simulink model "momentumBasedFlight"  (R2021b)
settings: Solver=VariableStepAuto  StartTime=0.0  StopTime=Config.simulationTime  RelTol=1e-3
InitFcn:
  | cd(fileparts(which(bdroot)));
  | initMomentumBasedFlight;
StopFcn:
  | cd(fileparts(which(bdroot)));
  | stopMomentumBasedFlight;
undefined symbols (not defined in the file or in its folder): aero_config, biasVectorConstraint_feet, Config, ConstraintMatrix_feet, DiscIntNeverNeededParam, frameNames, Frames
libraries: WBToolboxLibrary x104, momentum_flight_control_sublib x4, thrust_estimation_sublib x1, jets_control x1
(part 2 of 3)

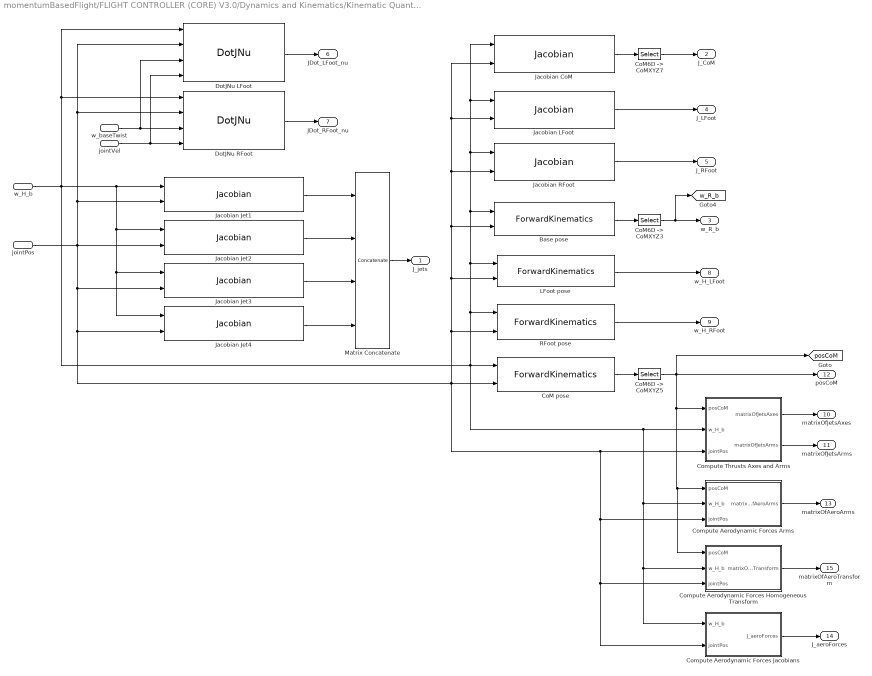
== system momentumBasedFlight/FLIGHT CONTROLLER (CORE) V3.0/Dynamics and Kinematics/Kinematic Quantities ==
  w_H_b : Inport
  jointPos : Inport  Port=2
  w_baseTwist : Inport  Port=3
  jointVel : Inport  Port=4
  Base pose : WBToolboxLibrary/Model/Kinematics/ForwardKinematics  frameName=Frames.BASE_LINK
      settings: SourceProductName=WholeBodyToolbox
  CoM pose : WBToolboxLibrary/Model/Kinematics/ForwardKinematics  frameName=Frames.COM_FRAME
      settings: SourceProductName=WholeBodyToolbox
  "CoM6D -> CoMXYZ3" : Selector  NumberOfDimensions=2  InputPortWidth=7  IndexOptions=Index vector (dialog),Index vector (dialog)  Indices=[1 2 3],[1 2 3]  OutputSizes=1,1
  "CoM6D -> CoMXYZ5" : Selector  NumberOfDimensions=2  InputPortWidth=7  IndexOptions=Index vector (dialog),Index vector (dialog)  Indices=[1 2 3],[4]  OutputSizes=1,1
  "CoM6D -> CoMXYZ7" : Selector  NumberOfDimensions=2  InputPortWidth=7  IndexOptions=Index vector (dialog),Index vector (dialog)  Indices=[1 2 3],[1:6+Config.N_DOF]  OutputSizes=1,1
  Compute Aerodynamic Forces Arms : Subsystem
  Compute Aerodynamic Forces Homogeneous Transform : Subsystem
  Compute Aerodynamic Forces Jacobians : Subsystem
  Compute Thrusts Axes and Arms : Subsystem
  DotJNu LFoot : WBToolboxLibrary/Model/Jacobians/DotJNu  frameName=Frames.LFOOT_FRAME
      settings: SourceProductName=WholeBodyToolbox
  DotJNu RFoot : WBToolboxLibrary/Model/Jacobians/DotJNu  frameName=Frames.RFOOT_FRAME
      settings: SourceProductName=WholeBodyToolbox
  Jacobian CoM : WBToolboxLibrary/Model/Jacobians/Jacobian  frameName=Frames.COM_FRAME
      settings: SourceProductName=WholeBodyToolbox
  Jacobian Jet1 : WBToolboxLibrary/Model/Jacobians/Jacobian  frameName=Frames.JET1_FRAME
      settings: SourceProductName=WholeBodyToolbox
  Jacobian Jet2 : WBToolboxLibrary/Model/Jacobians/Jacobian  frameName=Frames.JET2_FRAME
      settings: SourceProductName=WholeBodyToolbox
  Jacobian Jet3 : WBToolboxLibrary/Model/Jacobians/Jacobian  frameName=Frames.JET3_FRAME
      settings: SourceProductName=WholeBodyToolbox
  Jacobian Jet4 : WBToolboxLibrary/Model/Jacobians/Jacobian  frameName=Frames.JET4_FRAME
      settings: SourceProductName=WholeBodyToolbox
  Jacobian LFoot : WBToolboxLibrary/Model/Jacobians/Jacobian  frameName=Frames.LFOOT_FRAME
      settings: SourceProductName=WholeBodyToolbox
  Jacobian RFoot : WBToolboxLibrary/Model/Jacobians/Jacobian  frameName=Frames.RFOOT_FRAME
      settings: SourceProductName=WholeBodyToolbox
  LFoot pose : WBToolboxLibrary/Model/Kinematics/ForwardKinematics  frameName=Frames.LFOOT_FRAME
      settings: SourceProductName=WholeBodyToolbox
  Matrix Concatenate : Concatenate  NumInputs=4  Mode=Multidimensional array
  RFoot pose : WBToolboxLibrary/Model/Kinematics/ForwardKinematics  frameName=Frames.RFOOT_FRAME
      settings: SourceProductName=WholeBodyToolbox
  J_jets : Outport  VectorParamsAs1DForOutWhenUnconnected=off
  J_CoM : Outport  Port=2  VectorParamsAs1DForOutWhenUnconnected=off
  w_R_b : Outport  Port=3  VectorParamsAs1DForOutWhenUnconnected=off
  J_LFoot : Outport  Port=4  VectorParamsAs1DForOutWhenUnconnected=off
  J_RFoot : Outport  Port=5  VectorParamsAs1DForOutWhenUnconnected=off
  JDot_LFoot_nu : Outport  Port=6  VectorParamsAs1DForOutWhenUnconnected=off
  JDot_RFoot_nu : Outport  Port=7  VectorParamsAs1DForOutWhenUnconnected=off
  w_H_LFoot : Outport  Port=8  VectorParamsAs1DForOutWhenUnconnected=off
  w_H_RFoot : Outport  Port=9  VectorParamsAs1DForOutWhenUnconnected=off
  matrixOfJetsAxes : Outport  Port=10  VectorParamsAs1DForOutWhenUnconnected=off
  matrixOfJetsArms : Outport  Port=11  VectorParamsAs1DForOutWhenUnconnected=off
  posCoM : Outport  Port=12  VectorParamsAs1DForOutWhenUnconnected=off
  matrixOfAeroArms : Outport  Port=13
  J_aeroForces : Outport  Port=14
  matrixOfAeroTransform : Outport  Port=15
  tag scope: posCoM=global, w_R_b=global
  wires:
  "CoM6D -> CoMXYZ7"/1 -> J_CoM/1
  Jacobian Jet4/1 -> Matrix Concatenate/4
  Jacobian Jet3/1 -> Matrix Concatenate/3
  Jacobian Jet2/1 -> Matrix Concatenate/2
  Jacobian Jet1/1 -> Matrix Concatenate/1
  Compute Thrusts Axes and Arms/1(matrixOfJetsAxes) -> matrixOfJetsAxes/1
  Compute Thrusts Axes and Arms/2(matrixOfJetsArms) -> matrixOfJetsArms/1
  Base pose/1 -> "CoM6D -> CoMXYZ3"/1
  LFoot pose/1 -> w_H_LFoot/1
  RFoot pose/1 -> w_H_RFoot/1
  w_baseTwist/1 -> DotJNu RFoot/3, DotJNu LFoot/3
  jointVel/1 -> DotJNu LFoot/4, DotJNu RFoot/4
  DotJNu LFoot/1 -> JDot_LFoot_nu/1
  DotJNu RFoot/1 -> JDot_RFoot_nu/1
  Jacobian LFoot/1 -> J_LFoot/1
  Jacobian RFoot/1 -> J_RFoot/1
  Jacobian CoM/1 -> "CoM6D -> CoMXYZ7"/1
  jointPos/1 -> Jacobian Jet1/2, DotJNu RFoot/2, DotJNu LFoot/2, Jacobian Jet2/2, Base pose/2, Jacobian CoM/2, Jacobian LFoot/2, Jacobian RFoot/2, LFoot pose/2, RFoot pose/2, CoM pose/2, Compute Aerodynamic Forces Homogeneous Transform/3(jointPos), Compute Aerodynamic Forces Jacobians/2(jointPos), Compute Aerodynamic Forces Arms/3(jointPos), Compute Thrusts Axes and Arms/3(jointPos), Jacobian Jet4/2, Jacobian Jet3/2
  "CoM6D -> CoMXYZ3"/1 -> [w_R_b], w_R_b/1
  w_H_b/1 -> Jacobian Jet1/1, Jacobian Jet2/1, Jacobian Jet3/1, Jacobian Jet4/1, DotJNu RFoot/1, DotJNu LFoot/1, Compute Aerodynamic Forces Homogeneous Transform/2(w_H_b), Compute Aerodynamic Forces Jacobians/1(w_H_b), Compute Aerodynamic Forces Arms/2(w_H_b), Compute Thrusts Axes and Arms/2(w_H_b), CoM pose/1, RFoot pose/1, Jacobian RFoot/1, Jacobian CoM/1, Jacobian LFoot/1, Base pose/1, LFoot pose/1
  CoM pose/1 -> "CoM6D -> CoMXYZ5"/1
  Matrix Concatenate/1 -> J_jets/1
  "CoM6D -> CoMXYZ5"/1 -> Compute Aerodynamic Forces Homogeneous Transform/1(posCoM), Compute Aerodynamic Forces Arms/1(posCoM), Compute Thrusts Axes and Arms/1(posCoM), [posCoM], posCoM/1
  Compute Aerodynamic Forces Arms/1(matrixOfAeroArms) -> matrixOfAeroArms/1
  Compute Aerodynamic Forces Jacobians/1(J_aeroForces) -> J_aeroForces/1
  Compute Aerodynamic Forces Homogeneous Transform/1(matrixOfCoMTransform) -> matrixOfAeroTransform/1

== system momentumBasedFlight/FLIGHT CONTROLLER (CORE) V3.0/Estimated or Measured Thrusts/ Thrust Estimator ==
  w_H_b : Inport
  jointPos : Inport  Port=2
  dynamics : Inport  Port=3
  wrench_LFoot : Inport  Port=4
  wrench_RFoot : Inport  Port=5
  throttle : Inport  Port=6
  Enable : EnablePort
  Bus Selector : BusSelector  OutputSignals=L
  Constant : Constant  Value=0
  Constant1 : Constant
  EKF-MOMENTUM_JET_FEET-CMM_FEET : thrust_estimation_sublib/For Simulation/EKF-MOMENTUM_JET_FEET-CMM_FEET  Ts=Config.tStep  Frames=Frames  T0=[0.0; 0.0; 0.0; 0.0]  dot_T0=[0.0; 0.0; 0.0; 0.0]  h0=[0.0; 0.0; 0.0; 0.0; 0.0; 0.0]  fLF0=[0.0; 0.0; 200.0; 0.0; 0.0; 0.0]  fRF0=[0.0; 0.0; 200.0; 0.0; 0.0; 0.0]  P0=blkdiag(eye(4)*1e1, eye(4)*1e1, eye(6)*1e1, eye(6)*1e1, eye(6)*1e1)  Q=blkdiag(eye(4)*1e1, eye(4)*1e1, eye(6)*1e1, eye(6)*1e1, eye(6)*1e1)  R=blkdiag(eye(6)*1e1, eye(6)*1e1, eye(6)*1e1)  jetC_P100=Config.jetC_P100  jetC_P220=Config.jetC_P220
      settings: SourceProductName=iRonCub Library
  Manual Switch : ManualSwitch
  Terminator : Terminator
  Terminator1 : Terminator
  Terminator2 : Terminator
  Unit Delay : UnitDelay  SampleTime=-1  HasFrameUpgradeWarning=on
  jetIntensities_Estimated : Outport
  jetIntensitiesDot_Estimated : Outport  Port=2
  wires:
  Unit Delay/1 -> EKF-MOMENTUM_JET_FEET-CMM_FEET/1
  wrench_RFoot/1 -> EKF-MOMENTUM_JET_FEET-CMM_FEET/6
  wrench_LFoot/1 -> EKF-MOMENTUM_JET_FEET-CMM_FEET/5
  EKF-MOMENTUM_JET_FEET-CMM_FEET/5 -> Terminator2/1
  EKF-MOMENTUM_JET_FEET-CMM_FEET/4 -> Terminator1/1
  EKF-MOMENTUM_JET_FEET-CMM_FEET/3 -> Terminator/1
  jointPos/1 -> EKF-MOMENTUM_JET_FEET-CMM_FEET/2
  w_H_b/1 -> EKF-MOMENTUM_JET_FEET-CMM_FEET/3
  throttle/1 -> Unit Delay/1
  EKF-MOMENTUM_JET_FEET-CMM_FEET/2 -> jetIntensitiesDot_Estimated/1
  EKF-MOMENTUM_JET_FEET-CMM_FEET/1 -> jetIntensities_Estimated/1
  Bus Selector/1 -> EKF-MOMENTUM_JET_FEET-CMM_FEET/4  "<L>"
  dynamics/1 -> Bus Selector/1
  Manual Switch/1 -> EKF-MOMENTUM_JET_FEET-CMM_FEET/7
  Constant/1 -> Manual Switch/2
  Constant1/1 -> Manual Switch/1

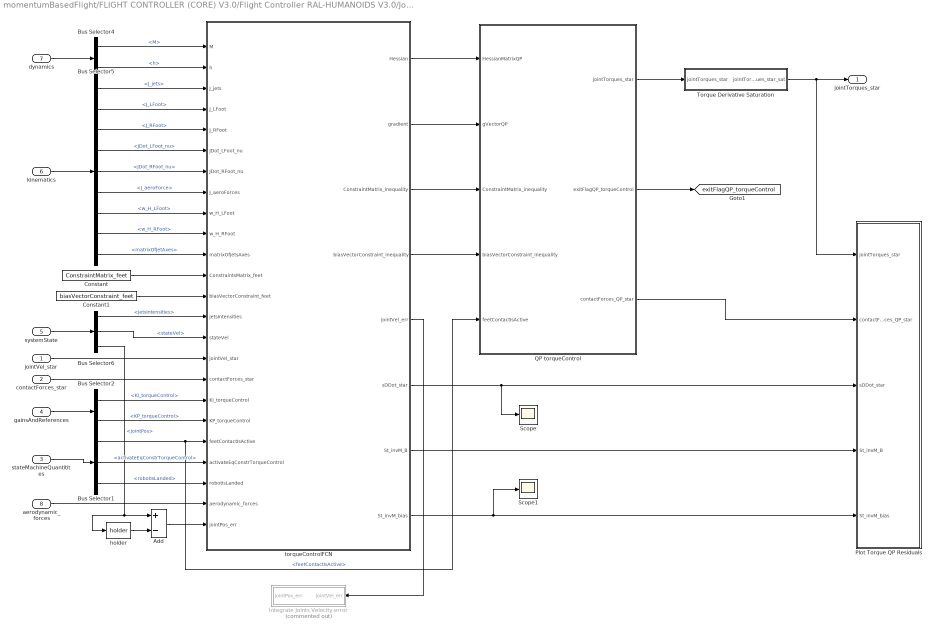
== system momentumBasedFlight/FLIGHT CONTROLLER (CORE) V3.0/Flight Controller RAL-HUMANOIDS V3.0/Joint Torque Control for Flying ==
  jointVel_star : Inport
  contactForces_star : Inport  Port=2
  stateMachineQuantitites : Inport  Port=3
  gainsAndReferences : Inport  Port=4
  systemState : Inport  Port=5
  kinematics : Inport  Port=6
  dynamics : Inport  Port=7
  aerodynamic_forces : Inport  Port=8
  Add : Sum  Inputs=+-
  Bus Selector1 : BusSelector  OutputSignals=feetContactIsActive,activateEqConstrTorqueControl,robotIsLanded
  Bus Selector2 : BusSelector  OutputSignals=KI_torqueControl,KP_torqueControl
  Bus Selector4 : BusSelector  OutputSignals=M,h
  Bus Selector5 : BusSelector  OutputSignals=J_jets,J_LFoot,J_RFoot,JDot_LFoot_nu,JDot_RFoot_nu,J_aeroForce,w_H_LFoot,w_H_RFoot,matrixOfJetAxes
  Bus Selector6 : BusSelector  OutputSignals=jetsIntensities,stateVel,jointPos
  Constant : Constant  Value=ConstraintMatrix_feet
  Constant1 : Constant  Value=biasVectorConstraint_feet
  Integrate Joints Velocity error : Subsystem  Commented=on
  Plot Torque QP Residuals : Subsystem
  QP torqueControl : Subsystem
  Scope : Scope
  Scope1 : Scope
  Torque Derivative Saturation : Subsystem
  "holder " : WBToolboxLibrary/Utilities/holder 
      settings: SourceProductName=WholeBodyToolbox
  torqueControlFCN : MATLAB Function  TreatAsAtomicUnit=on
  jointTorques_star : Outport  VectorParamsAs1DForOutWhenUnconnected=off
  tag scope: exitFlagQP_torqueControl=global
  wires:
  Torque Derivative Saturation/1(jointTorques_star_sat) -> Plot Torque QP Residuals/1(jointTorques_star), jointTorques_star/1
  Bus Selector1/2 -> torqueControlFCN/21(activateEqConstrTorqueControl)  "<activateEqConstrTorqueControl>"
  Bus Selector1/3 -> torqueControlFCN/22(robotIsLanded)  "<robotIsLanded>"
  torqueControlFCN/5(jointVel_err) -> Integrate Joints Velocity error/1(jointVel_err)
  Bus Selector5/9 -> torqueControlFCN/11(matrixOfJetsAxes)  "<matrixOfJetAxes>"
  jointVel_star/1 -> torqueControlFCN/16(jointVel_star)
  torqueControlFCN/4(biasVectorConstraint_inequality) -> QP torqueControl/4(biasVectorConstraint_inequality)
  torqueControlFCN/3(ConstraintMatrix_inequality) -> QP torqueControl/3(ConstraintMatrix_inequality)
  torqueControlFCN/2(gradient) -> QP torqueControl/2(gVectorQP)
  torqueControlFCN/1(Hessian) -> QP torqueControl/1(HessianMatrixQP)
  Bus Selector2/2 -> torqueControlFCN/19(KP_torqueControl)  "<KP_torqueControl>"
  Bus Selector2/1 -> torqueControlFCN/18(KI_torqueControl)  "<KI_torqueControl>"
  gainsAndReferences/1 -> Bus Selector2/1
  Bus Selector1/1 -> QP torqueControl/5(feetContactIsActive), torqueControlFCN/20(feetContactIsActive)  "<feetContactIsActive>"
  stateMachineQuantitites/1 -> Bus Selector1/1
  Bus Selector6/1 -> torqueControlFCN/14(jetsIntensities)  "<jetsIntensities>"
  QP torqueControl/2(exitFlagQP_torqueControl) -> [exitFlagQP_torqueControl]
  QP torqueControl/1(jointTorques_star) -> Torque Derivative Saturation/1(jointTorques_star)
  contactForces_star/1 -> torqueControlFCN/17(contactForces_star)
  Constant/1 -> torqueControlFCN/12(ConstraintsMatrix_feet)
  Constant1/1 -> torqueControlFCN/13(biasVectorConstraint_feet)
  Bus Selector5/8 -> torqueControlFCN/10(w_H_RFoot)  "<w_H_RFoot>"
  Bus Selector5/7 -> torqueControlFCN/9(w_H_LFoot)  "<w_H_LFoot>"
  Bus Selector5/5 -> torqueControlFCN/7(JDot_RFoot_nu)  "<JDot_RFoot_nu>"
  Bus Selector5/4 -> torqueControlFCN/6(JDot_LFoot_nu)  "<JDot_LFoot_nu>"
  Bus Selector5/3 -> torqueControlFCN/5(J_RFoot)  "<J_RFoot>"
  Bus Selector5/2 -> torqueControlFCN/4(J_LFoot)  "<J_LFoot>"
  Bus Selector5/1 -> torqueControlFCN/3(J_jets)  "<J_jets>"
  Bus Selector4/2 -> torqueControlFCN/2(h)  "<h>"
  Bus Selector4/1 -> torqueControlFCN/1(M)  "<M>"
  kinematics/1 -> Bus Selector5/1
  systemState/1 -> Bus Selector6/1
  dynamics/1 -> Bus Selector4/1
  Bus Selector6/2 -> torqueControlFCN/15(stateVel)  "<stateVel>"
  Bus Selector5/6 -> torqueControlFCN/8(J_aeroForces)  "<J_aeroForce>"
  aerodynamic_forces/1 -> torqueControlFCN/23(aerodynamic_forces)
  Bus Selector6/3 -> "holder "/1, Add/1  "<jointPos>"
  Add/1 -> torqueControlFCN/24(jointPos_err)
  "holder "/1 -> Add/2
  QP torqueControl/3(contactForces_QP_star) -> Plot Torque QP Residuals/2(contactForces_QP_star)
  torqueControlFCN/6(sDDot_star) -> Scope/1, Plot Torque QP Residuals/3(sDDot_star)
  torqueControlFCN/7(St_invM_B) -> Plot Torque QP Residuals/4(St_invM_B)
  torqueControlFCN/8(St_invM_bias) -> Scope1/1, Plot Torque QP Residuals/5(St_invM_bias)

== system momentumBasedFlight/FLIGHT CONTROLLER (CORE) V3.0/Flight Controller RAL-HUMANOIDS V3.0/Momentum Control for Flying ==
  stateMachineQuantitites : Inport
  gainsAndReferences : Inport  Port=2
  systemState : Inport  Port=3
  kinematics : Inport  Port=4
  dynamics : Inport  Port=5
  aerodynamic_forces : Inport  Port=6
  Momentum Control : Subsystem
  QP Solver and Integrate Contact Forces Derivative : Subsystem
  jointVel_star : Outport  VectorParamsAs1DForOutWhenUnconnected=off
  contactForces_star : Outport  Port=2  VectorParamsAs1DForOutWhenUnconnected=off
  jetsIntensitiesDot_star : Outport  Port=3  VectorParamsAs1DForOutWhenUnconnected=off
  wires:
  QP Solver and Integrate Contact Forces Derivative/3(jointVel_star) -> jointVel_star/1
  QP Solver and Integrate Contact Forces Derivative/1(contactForces_star) -> Momentum Control/1(contactForces_hat), contactForces_star/1  "WARNING! estimated contact forces are assumed to be coincident with contactForces_star"
  Momentum Control/4(uppeBoundQP) -> QP Solver and Integrate Contact Forces Derivative/4(upperBoundQP)
  Momentum Control/3(lowerBoundQP) -> QP Solver and Integrate Contact Forces Derivative/3(lowerBoundQP)
  Momentum Control/2(gVectorQP) -> QP Solver and Integrate Contact Forces Derivative/2(gVectorQP)
  Momentum Control/1(HessianMatrixQP) -> QP Solver and Integrate Contact Forces Derivative/1(HessianMatrixQP)
  stateMachineQuantitites/1 -> QP Solver and Integrate Contact Forces Derivative/5(stateMachineQuantities), Momentum Control/6(stateMachineQuantitites)
  gainsAndReferences/1 -> Momentum Control/5(gainsAndReferences)
  dynamics/1 -> Momentum Control/4(dynamics), QP Solver and Integrate Contact Forces Derivative/7(dynamics)
  kinematics/1 -> Momentum Control/3(kinematics)
  systemState/1 -> QP Solver and Integrate Contact Forces Derivative/6(systemState), Momentum Control/2(systemState)
  QP Solver and Integrate Contact Forces Derivative/2(jetsIntensitiesDot_star) -> jetsIntensitiesDot_star/1
  aerodynamic_forces/1 -> Momentum Control/7(aerodynamic_forces)

== system momentumBasedFlight/FLIGHT CONTROLLER (CORE) V3.0/Flight Controller RAL-HUMANOIDS V3.0/deadZone ==
  u : Inport
  Constant : Constant  Value=Config.sat.deadZoneThresholdJointVel
  Deadzone Function : MATLAB Function  TreatAsAtomicUnit=on
  u_cut : Outport  VectorParamsAs1DForOutWhenUnconnected=off
  wires:
  Constant/1 -> Deadzone Function/2(thr)
  u/1 -> Deadzone Function/1(u)
  Deadzone Function/1(y) -> u_cut/1

== system momentumBasedFlight/FLOATING BASE ESTIMATOR/Compute State Velocity/Feet Jacobians ==
  jointPos : Inport
  w_H_b : Inport  Port=2
  Jacobian l_sole : WBToolboxLibrary/Model/Jacobians/Jacobian  frameName=Frames.LFOOT_FRAME
      settings: SourceProductName=WholeBodyToolbox
  Jacobian r_sole : WBToolboxLibrary/Model/Jacobians/Jacobian  frameName=Frames.RFOOT_FRAME
      settings: SourceProductName=WholeBodyToolbox
  J_l_sole : Outport  VectorParamsAs1DForOutWhenUnconnected=off
  J_r_sole : Outport  Port=2  VectorParamsAs1DForOutWhenUnconnected=off
  wires:
  Jacobian l_sole/1 -> J_l_sole/1
  Jacobian r_sole/1 -> J_r_sole/1
  w_H_b/1 -> Jacobian r_sole/1, Jacobian l_sole/1
  jointPos/1 -> Jacobian l_sole/2, Jacobian r_sole/2

== system momentumBasedFlight/FLOATING BASE ESTIMATOR/Compute base to fixed link transform/LFoot to base link transform  ==
  jointPos : Inport
  inertial : Inport  Port=2
  w_H_link : Inport  Port=3
  w_H_base_fixed : Inport  Port=4
  Fixed base to imu transform : WBToolboxLibrary/Model/Kinematics/ForwardKinematics  frameName=Frames.IMU
      settings: SourceProductName=WholeBodyToolbox
  Fixed base to root link transform : WBToolboxLibrary/Model/Kinematics/ForwardKinematics  frameName=Frames.BASE_LINK
      settings: SourceProductName=WholeBodyToolbox
  Get Base Rotation From IMU : MATLAB Function  TreatAsAtomicUnit=on
  Inv : Product  Inputs=/*  Multiplication=Matrix(*)
  Inv_2 : Product  Inputs=/*  Multiplication=Matrix(*)
  Neck Position : WBToolboxLibrary/Utilities/YarpRead  portName=Ports.NECK_POS  signalSize=Ports.NECK_POS_PORT_SIZE  timeout=0.5  blocking=off  timestamp=off  autoconnect=on  errorOnConnection=off
      settings: SourceProductName=WholeBodyToolbox
  Selector1 : Selector  InputPortWidth=Ports.IMU_PORT_SIZE  IndexOptions=Index vector (dialog)  Indices=Ports.IMU_PORT_ORIENTATION_INDEX  OutputSizes=1
  Selector2 : Selector  InputPortWidth=Ports.IMU_PORT_SIZE  IndexOptions=Index vector (dialog)  Indices=Ports.IMU_PORT_ORIENTATION_INDEX  OutputSizes=1
  Switch6 : Switch  Criteria=u2 > Threshold
  USE_IMU4EST_BASE : Constant  Value=Config.USE_IMU4EST_BASE
  holder 1 : WBToolboxLibrary/Utilities/holder 
      settings: SourceProductName=WholeBodyToolbox
  holder 2 : WBToolboxLibrary/Utilities/holder 
      settings: SourceProductName=WholeBodyToolbox
  neck transform : Subsystem
  link_H_b : Outport  VectorParamsAs1DForOutWhenUnconnected=off
  wires:
  Switch6/1 -> link_H_b/1
  Inv_2/1 -> Switch6/3, Get Base Rotation From IMU/3(fixedLink_H_base)  "link_H_root"
  USE_IMU4EST_BASE/1 -> Switch6/2
  Inv/1 -> Get Base Rotation From IMU/1(imu_H_fixedLink), holder 1/1  "imu_H_link"
  holder 2/1 -> Selector2/1
  Fixed base to imu transform/1 -> Inv/1
  jointPos/1 -> Fixed base to imu transform/2, Fixed base to root link transform/2
  Get Base Rotation From IMU/1(w_H_b) -> Switch6/1
  Fixed base to root link transform/1 -> Inv_2/2
  inertial/1 -> holder 2/1, Selector1/1
  Neck Position/1 -> neck transform/1(neck port)
  neck transform/1(neck position) -> Get Base Rotation From IMU/6(neck_pos)
  w_H_link/1 -> Inv_2/1, Inv/2
  w_H_base_fixed/1 -> Fixed base to root link transform/1, Fixed base to imu transform/1
  Selector2/1 -> Get Base Rotation From IMU/4(rpyFromIMU_0)
  holder 1/1 -> Get Base Rotation From IMU/2(imu_H_fixedLink_0)
  Selector1/1 -> Get Base Rotation From IMU/5(rpyFromIMU)

== system momentumBasedFlight/FLOATING BASE ESTIMATOR/Compute base to fixed link transform/RFoot to base link transform ==
  jointPos : Inport
  inertial : Inport  Port=2
  w_H_link : Inport  Port=3
  w_H_base_fixed : Inport  Port=4
  Fixed base to imu transform : WBToolboxLibrary/Model/Kinematics/ForwardKinematics  frameName=Frames.IMU
      settings: SourceProductName=WholeBodyToolbox
  Fixed base to root link transform : WBToolboxLibrary/Model/Kinematics/ForwardKinematics  frameName=Frames.BASE_LINK
      settings: SourceProductName=WholeBodyToolbox
  Get Base Rotation From IMU : MATLAB Function  TreatAsAtomicUnit=on
  Inv : Product  Inputs=/*  Multiplication=Matrix(*)
  Inv_2 : Product  Inputs=/*  Multiplication=Matrix(*)
  Neck Position : WBToolboxLibrary/Utilities/YarpRead  portName=Ports.NECK_POS  signalSize=Ports.NECK_POS_PORT_SIZE  timeout=0.5  blocking=off  timestamp=off  autoconnect=on  errorOnConnection=off
      settings: SourceProductName=WholeBodyToolbox
  Selector1 : Selector  InputPortWidth=Ports.IMU_PORT_SIZE  IndexOptions=Index vector (dialog)  Indices=Ports.IMU_PORT_ORIENTATION_INDEX  OutputSizes=1
  Selector2 : Selector  InputPortWidth=Ports.IMU_PORT_SIZE  IndexOptions=Index vector (dialog)  Indices=Ports.IMU_PORT_ORIENTATION_INDEX  OutputSizes=1
  Switch6 : Switch  Criteria=u2 > Threshold
  USE_IMU4EST_BASE : Constant  Value=Config.USE_IMU4EST_BASE
  holder 1 : WBToolboxLibrary/Utilities/holder 
      settings: SourceProductName=WholeBodyToolbox
  holder 2 : WBToolboxLibrary/Utilities/holder 
      settings: SourceProductName=WholeBodyToolbox
  neck transform : Subsystem
  link_H_b : Outport  VectorParamsAs1DForOutWhenUnconnected=off
  wires:
  Switch6/1 -> link_H_b/1
  Inv_2/1 -> Switch6/3, Get Base Rotation From IMU/3(fixedLink_H_base)  "link_H_root"
  USE_IMU4EST_BASE/1 -> Switch6/2
  Inv/1 -> Get Base Rotation From IMU/1(imu_H_fixedLink), holder 1/1  "imu_H_link"
  holder 2/1 -> Selector2/1
  Fixed base to imu transform/1 -> Inv/1
  jointPos/1 -> Fixed base to imu transform/2, Fixed base to root link transform/2
  Get Base Rotation From IMU/1(w_H_b) -> Switch6/1
  Fixed base to root link transform/1 -> Inv_2/2
  inertial/1 -> holder 2/1, Selector1/1
  Neck Position/1 -> neck transform/1(neck port)
  neck transform/1(neck position) -> Get Base Rotation From IMU/6(neck_pos)
  w_H_link/1 -> Inv_2/1, Inv/2
  w_H_base_fixed/1 -> Fixed base to root link transform/1, Fixed base to imu transform/1
  Selector2/1 -> Get Base Rotation From IMU/4(rpyFromIMU_0)
  holder 1/1 -> Get Base Rotation From IMU/2(imu_H_fixedLink_0)
  Selector1/1 -> Get Base Rotation From IMU/5(rpyFromIMU)

== system momentumBasedFlight/Visualizer/Task and Base Frame Kinematics/Combine Rotations ==
  roll : Inport
  pitch : Inport  Port=2
  yaw : Inport  Port=3
  roll_des : Inport  Port=4
  pitch_des : Inport  Port=5
  yaw_des : Inport  Port=6
  Mux : Mux  Inputs=2
  Mux1 : Mux  Inputs=2
  Mux2 : Mux  Inputs=2
  Task rotation combined : Scope  NumInputPorts=3
  wires:
  yaw_des/1 -> Mux2/2
  pitch_des/1 -> Mux1/2
  pitch/1 -> Mux1/1
  roll/1 -> Mux/1
  yaw/1 -> Mux2/1
  roll_des/1 -> Mux/2
  Mux2/1 -> Task rotation combined/3
  Mux1/1 -> Task rotation combined/2
  Mux/1 -> Task rotation combined/1

== system momentumBasedFlight/FLIGHT CONTROLLER (CORE) V3.0/Dynamics and Kinematics/Dynamic Quantities/Compute Centroidal Inertia ==
  M : Inport
  w_H_b : Inport  Port=2
  posCoM : Inport  Port=3
  Compute Centroidal Inertia : MATLAB Function  TreatAsAtomicUnit=on
  Selector : Selector  NumberOfDimensions=2  InputPortWidth=3  IndexOptions=Index vector (dialog),Index vector (dialog)  Indices=[1 2 3],4  OutputSizes=1,1
  w_I_c : Outport  VectorParamsAs1DForOutWhenUnconnected=off
  wires:
  Compute Centroidal Inertia/1(w_I_c) -> w_I_c/1
  posCoM/1 -> Compute Centroidal Inertia/2(posCoM)
  Selector/1 -> Compute Centroidal Inertia/3(posBase)
  w_H_b/1 -> Selector/1
  M/1 -> Compute Centroidal Inertia/1(M)

== system momentumBasedFlight/FLIGHT CONTROLLER (CORE) V3.0/Dynamics and Kinematics/Dynamic Quantities/Momentum and CentroidalMomentum Matrix ==
  w_H_b : Inport
  jointPos : Inport  Port=2
  w_baseTwist : Inport  Port=3
  jointVel : Inport  Port=4
  CentroidalMomentum : WBToolboxLibrary/Model/Dynamics/CentroidalMomentum
      settings: SourceProductName=WholeBodyToolbox
  CentroidalTotalMomentumMatrix : WBToolboxLibrary/Model/Jacobians/CentroidalTotalMomentumMatrix
      settings: SourceProductName=WholeBodyToolbox
  L : Outport  VectorParamsAs1DForOutWhenUnconnected=off
  CMM : Outport  Port=2  VectorParamsAs1DForOutWhenUnconnected=off
  wires:
  CentroidalTotalMomentumMatrix/1 -> CMM/1
  jointVel/1 -> CentroidalMomentum/4
  jointPos/1 -> CentroidalMomentum/2, CentroidalTotalMomentumMatrix/2
  w_H_b/1 -> CentroidalMomentum/1, CentroidalTotalMomentumMatrix/1
  CentroidalMomentum/1 -> L/1
  w_baseTwist/1 -> CentroidalMomentum/3

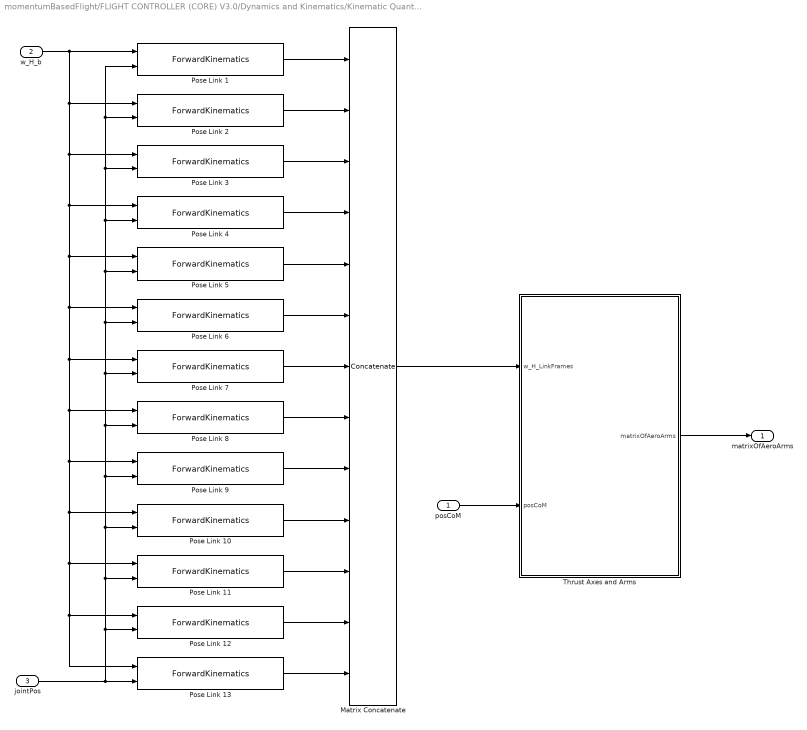
== system momentumBasedFlight/FLIGHT CONTROLLER (CORE) V3.0/Dynamics and Kinematics/Kinematic Quantities/Compute Aerodynamic Forces Arms ==
  posCoM : Inport
  w_H_b : Inport  Port=2
  jointPos : Inport  Port=3
  Matrix Concatenate : Concatenate  NumInputs=13  Mode=Multidimensional array  ConcatenateDimension=2
  Pose Link 1 : WBToolboxLibrary/Model/Kinematics/ForwardKinematics  frameName=frameNames{1}
      settings: SourceProductName=WholeBodyToolbox
  Pose Link 10 : WBToolboxLibrary/Model/Kinematics/ForwardKinematics  frameName=frameNames{10}
      settings: SourceProductName=WholeBodyToolbox
  Pose Link 11 : WBToolboxLibrary/Model/Kinematics/ForwardKinematics  frameName=frameNames{11}
      settings: SourceProductName=WholeBodyToolbox
  Pose Link 12 : WBToolboxLibrary/Model/Kinematics/ForwardKinematics  frameName=frameNames{12}
      settings: SourceProductName=WholeBodyToolbox
  Pose Link 13 : WBToolboxLibrary/Model/Kinematics/ForwardKinematics  frameName=frameNames{13}
      settings: SourceProductName=WholeBodyToolbox
  Pose Link 2 : WBToolboxLibrary/Model/Kinematics/ForwardKinematics  frameName=frameNames{2}
      settings: SourceProductName=WholeBodyToolbox
  Pose Link 3 : WBToolboxLibrary/Model/Kinematics/ForwardKinematics  frameName=frameNames{3}
      settings: SourceProductName=WholeBodyToolbox
  Pose Link 4 : WBToolboxLibrary/Model/Kinematics/ForwardKinematics  frameName=frameNames{4}
      settings: SourceProductName=WholeBodyToolbox
  Pose Link 5 : WBToolboxLibrary/Model/Kinematics/ForwardKinematics  frameName=frameNames{5}
      settings: SourceProductName=WholeBodyToolbox
  Pose Link 6 : WBToolboxLibrary/Model/Kinematics/ForwardKinematics  frameName=frameNames{6}
      settings: SourceProductName=WholeBodyToolbox
  Pose Link 7 : WBToolboxLibrary/Model/Kinematics/ForwardKinematics  frameName=frameNames{7}
      settings: SourceProductName=WholeBodyToolbox
  Pose Link 8 : WBToolboxLibrary/Model/Kinematics/ForwardKinematics  frameName=frameNames{8}
      settings: SourceProductName=WholeBodyToolbox
  Pose Link 9 : WBToolboxLibrary/Model/Kinematics/ForwardKinematics  frameName=frameNames{9}
      settings: SourceProductName=WholeBodyToolbox
  Thrust Axes and Arms : MATLAB Function  TreatAsAtomicUnit=on
  matrixOfAeroArms : Outport  VectorParamsAs1DForOutWhenUnconnected=off
  wires:
  posCoM/1 -> Thrust Axes and Arms/2(posCoM)
  w_H_b/1 -> Pose Link 1/1, Pose Link 4/1, Pose Link 5/1, Pose Link 6/1, Pose Link 7/1, Pose Link 9/1, Pose Link 10/1, Pose Link 11/1, Pose Link 12/1, Pose Link 13/1, Pose Link 8/1, Pose Link 3/1, Pose Link 2/1
  Thrust Axes and Arms/1(matrixOfAeroArms) -> matrixOfAeroArms/1
  jointPos/1 -> Pose Link 13/2, Pose Link 12/2, Pose Link 11/2, Pose Link 10/2, Pose Link 9/2, Pose Link 8/2, Pose Link 7/2, Pose Link 6/2, Pose Link 5/2, Pose Link 4/2, Pose Link 3/2, Pose Link 2/2, Pose Link 1/2
  Matrix Concatenate/1 -> Thrust Axes and Arms/1(w_H_LinkFrames)
  Pose Link 13/1 -> Matrix Concatenate/13
  Pose Link 12/1 -> Matrix Concatenate/12
  Pose Link 11/1 -> Matrix Concatenate/11
  Pose Link 10/1 -> Matrix Concatenate/10
  Pose Link 9/1 -> Matrix Concatenate/9
  Pose Link 8/1 -> Matrix Concatenate/8
  Pose Link 7/1 -> Matrix Concatenate/7
  Pose Link 6/1 -> Matrix Concatenate/6
  Pose Link 5/1 -> Matrix Concatenate/5
  Pose Link 4/1 -> Matrix Concatenate/4
  Pose Link 3/1 -> Matrix Concatenate/3
  Pose Link 2/1 -> Matrix Concatenate/2
  Pose Link 1/1 -> Matrix Concatenate/1

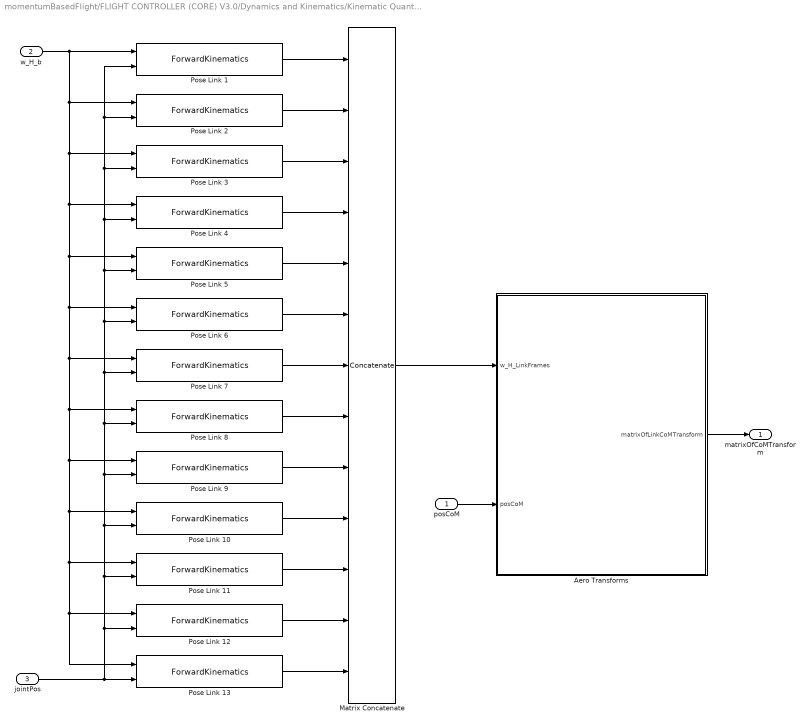
== system momentumBasedFlight/FLIGHT CONTROLLER (CORE) V3.0/Dynamics and Kinematics/Kinematic Quantities/Compute Aerodynamic Forces Homogeneous Transform ==
  posCoM : Inport
  w_H_b : Inport  Port=2
  jointPos : Inport  Port=3
  Aero Transforms : MATLAB Function  TreatAsAtomicUnit=on
  Matrix Concatenate : Concatenate  NumInputs=13  Mode=Multidimensional array  ConcatenateDimension=2
  Pose Link 1 : WBToolboxLibrary/Model/Kinematics/ForwardKinematics  frameName=frameNames{1}
      settings: SourceProductName=WholeBodyToolbox
  Pose Link 10 : WBToolboxLibrary/Model/Kinematics/ForwardKinematics  frameName=frameNames{10}
      settings: SourceProductName=WholeBodyToolbox
  Pose Link 11 : WBToolboxLibrary/Model/Kinematics/ForwardKinematics  frameName=frameNames{11}
      settings: SourceProductName=WholeBodyToolbox
  Pose Link 12 : WBToolboxLibrary/Model/Kinematics/ForwardKinematics  frameName=frameNames{12}
      settings: SourceProductName=WholeBodyToolbox
  Pose Link 13 : WBToolboxLibrary/Model/Kinematics/ForwardKinematics  frameName=frameNames{13}
      settings: SourceProductName=WholeBodyToolbox
  Pose Link 2 : WBToolboxLibrary/Model/Kinematics/ForwardKinematics  frameName=frameNames{2}
      settings: SourceProductName=WholeBodyToolbox
  Pose Link 3 : WBToolboxLibrary/Model/Kinematics/ForwardKinematics  frameName=frameNames{3}
      settings: SourceProductName=WholeBodyToolbox
  Pose Link 4 : WBToolboxLibrary/Model/Kinematics/ForwardKinematics  frameName=frameNames{4}
      settings: SourceProductName=WholeBodyToolbox
  Pose Link 5 : WBToolboxLibrary/Model/Kinematics/ForwardKinematics  frameName=frameNames{5}
      settings: SourceProductName=WholeBodyToolbox
  Pose Link 6 : WBToolboxLibrary/Model/Kinematics/ForwardKinematics  frameName=frameNames{6}
      settings: SourceProductName=WholeBodyToolbox
  Pose Link 7 : WBToolboxLibrary/Model/Kinematics/ForwardKinematics  frameName=frameNames{7}
      settings: SourceProductName=WholeBodyToolbox
  Pose Link 8 : WBToolboxLibrary/Model/Kinematics/ForwardKinematics  frameName=frameNames{8}
      settings: SourceProductName=WholeBodyToolbox
  Pose Link 9 : WBToolboxLibrary/Model/Kinematics/ForwardKinematics  frameName=frameNames{9}
      settings: SourceProductName=WholeBodyToolbox
  matrixOfCoMTransform : Outport  VectorParamsAs1DForOutWhenUnconnected=off
  wires:
  posCoM/1 -> Aero Transforms/2(posCoM)
  w_H_b/1 -> Pose Link 1/1, Pose Link 4/1, Pose Link 5/1, Pose Link 6/1, Pose Link 7/1, Pose Link 9/1, Pose Link 10/1, Pose Link 11/1, Pose Link 12/1, Pose Link 13/1, Pose Link 8/1, Pose Link 3/1, Pose Link 2/1
  Aero Transforms/1(matrixOfLinkCoMTransform) -> matrixOfCoMTransform/1
  jointPos/1 -> Pose Link 13/2, Pose Link 12/2, Pose Link 11/2, Pose Link 10/2, Pose Link 9/2, Pose Link 8/2, Pose Link 7/2, Pose Link 6/2, Pose Link 5/2, Pose Link 4/2, Pose Link 3/2, Pose Link 2/2, Pose Link 1/2
  Matrix Concatenate/1 -> Aero Transforms/1(w_H_LinkFrames)
  Pose Link 13/1 -> Matrix Concatenate/13
  Pose Link 12/1 -> Matrix Concatenate/12
  Pose Link 11/1 -> Matrix Concatenate/11
  Pose Link 10/1 -> Matrix Concatenate/10
  Pose Link 9/1 -> Matrix Concatenate/9
  Pose Link 8/1 -> Matrix Concatenate/8
  Pose Link 7/1 -> Matrix Concatenate/7
  Pose Link 6/1 -> Matrix Concatenate/6
  Pose Link 5/1 -> Matrix Concatenate/5
  Pose Link 4/1 -> Matrix Concatenate/4
  Pose Link 3/1 -> Matrix Concatenate/3
  Pose Link 2/1 -> Matrix Concatenate/2
  Pose Link 1/1 -> Matrix Concatenate/1

== system momentumBasedFlight/FLIGHT CONTROLLER (CORE) V3.0/Dynamics and Kinematics/Kinematic Quantities/Compute Aerodynamic Forces Jacobians ==
  w_H_b : Inport
  jointPos : Inport  Port=2
  Jacobian Link frame 1 : WBToolboxLibrary/Model/Jacobians/Jacobian  frameName=frameNames{1}
      settings: SourceProductName=WholeBodyToolbox
  Jacobian Link frame 10 : WBToolboxLibrary/Model/Jacobians/Jacobian  frameName=frameNames{10}
      settings: SourceProductName=WholeBodyToolbox
  Jacobian Link frame 11 : WBToolboxLibrary/Model/Jacobians/Jacobian  frameName=frameNames{11}
      settings: SourceProductName=WholeBodyToolbox
  Jacobian Link frame 12 : WBToolboxLibrary/Model/Jacobians/Jacobian  frameName=frameNames{12}
      settings: SourceProductName=WholeBodyToolbox
  Jacobian Link frame 13 : WBToolboxLibrary/Model/Jacobians/Jacobian  frameName=frameNames{13}
      settings: SourceProductName=WholeBodyToolbox
  Jacobian Link frame 2 : WBToolboxLibrary/Model/Jacobians/Jacobian  frameName=frameNames{2}
      settings: SourceProductName=WholeBodyToolbox
  Jacobian Link frame 3 : WBToolboxLibrary/Model/Jacobians/Jacobian  frameName=frameNames{3}
      settings: SourceProductName=WholeBodyToolbox
  Jacobian Link frame 4 : WBToolboxLibrary/Model/Jacobians/Jacobian  frameName=frameNames{4}
      settings: SourceProductName=WholeBodyToolbox
  Jacobian Link frame 5 : WBToolboxLibrary/Model/Jacobians/Jacobian  frameName=frameNames{5}
      settings: SourceProductName=WholeBodyToolbox
  Jacobian Link frame 6 : WBToolboxLibrary/Model/Jacobians/Jacobian  frameName=frameNames{6}
      settings: SourceProductName=WholeBodyToolbox
  Jacobian Link frame 7 : WBToolboxLibrary/Model/Jacobians/Jacobian  frameName=frameNames{7}
      settings: SourceProductName=WholeBodyToolbox
  Jacobian Link frame 8 : WBToolboxLibrary/Model/Jacobians/Jacobian  frameName=frameNames{8}
      settings: SourceProductName=WholeBodyToolbox
  Jacobian Link frame 9 : WBToolboxLibrary/Model/Jacobians/Jacobian  frameName=frameNames{9}
      settings: SourceProductName=WholeBodyToolbox
  Matrix Concatenate : Concatenate  NumInputs=13  Mode=Multidimensional array
  compute matrix of link CoM Jacobians : MATLAB Function  TreatAsAtomicUnit=on
  J_aeroForces : Outport  VectorParamsAs1DForOutWhenUnconnected=off
  wires:
  w_H_b/1 -> Jacobian Link frame 1/1, Jacobian Link frame 2/1, Jacobian Link frame 3/1, Jacobian Link frame 4/1, Jacobian Link frame 5/1, Jacobian Link frame 6/1, Jacobian Link frame 7/1, Jacobian Link frame 8/1, Jacobian Link frame 9/1, Jacobian Link frame 10/1, Jacobian Link frame 11/1, Jacobian Link frame 13/1, Jacobian Link frame 12/1, compute matrix of link CoM Jacobians/1(w_H_b)
  jointPos/1 -> Jacobian Link frame 13/2, Jacobian Link frame 12/2, Jacobian Link frame 11/2, Jacobian Link frame 10/2, Jacobian Link frame 9/2, Jacobian Link frame 8/2, Jacobian Link frame 7/2, Jacobian Link frame 6/2, Jacobian Link frame 5/2, Jacobian Link frame 4/2, Jacobian Link frame 3/2, Jacobian Link frame 1/2, Jacobian Link frame 2/2
  Jacobian Link frame 1/1 -> Matrix Concatenate/1
  Jacobian Link frame 2/1 -> Matrix Concatenate/2
  Jacobian Link frame 3/1 -> Matrix Concatenate/3
  Jacobian Link frame 5/1 -> Matrix Concatenate/5
  Jacobian Link frame 4/1 -> Matrix Concatenate/4
  Jacobian Link frame 6/1 -> Matrix Concatenate/6
  Jacobian Link frame 7/1 -> Matrix Concatenate/7
  Jacobian Link frame 8/1 -> Matrix Concatenate/8
  Jacobian Link frame 9/1 -> Matrix Concatenate/9
  Jacobian Link frame 10/1 -> Matrix Concatenate/10
  Jacobian Link frame 11/1 -> Matrix Concatenate/11
  Jacobian Link frame 12/1 -> Matrix Concatenate/12
  Jacobian Link frame 13/1 -> Matrix Concatenate/13
  compute matrix of link CoM Jacobians/1(J_aeroForces) -> J_aeroForces/1
  Matrix Concatenate/1 -> compute matrix of link CoM Jacobians/2(linkFrameJacobians)

== system momentumBasedFlight/FLIGHT CONTROLLER (CORE) V3.0/Dynamics and Kinematics/Kinematic Quantities/Compute Thrusts Axes and Arms ==
  posCoM : Inport
  w_H_b : Inport  Port=2
  jointPos : Inport  Port=3
  Pose Jet 1 : WBToolboxLibrary/Model/Kinematics/ForwardKinematics  frameName=Frames.JET1_FRAME
      settings: SourceProductName=WholeBodyToolbox
  Pose Jet 2 : WBToolboxLibrary/Model/Kinematics/ForwardKinematics  frameName=Frames.JET2_FRAME
      settings: SourceProductName=WholeBodyToolbox
  Pose Jet 3 : WBToolboxLibrary/Model/Kinematics/ForwardKinematics  frameName=Frames.JET3_FRAME
      settings: SourceProductName=WholeBodyToolbox
  Pose Jet 4 : WBToolboxLibrary/Model/Kinematics/ForwardKinematics  frameName=Frames.JET4_FRAME
      settings: SourceProductName=WholeBodyToolbox
  Thrust Axes and Arms : MATLAB Function  TreatAsAtomicUnit=on
  matrixOfJetsAxes : Outport  VectorParamsAs1DForOutWhenUnconnected=off
  matrixOfJetsArms : Outport  Port=2  VectorParamsAs1DForOutWhenUnconnected=off
  wires:
  posCoM/1 -> Thrust Axes and Arms/5(posCoM)
  w_H_b/1 -> Pose Jet 1/1, Pose Jet 2/1, Pose Jet 3/1, Pose Jet 4/1
  Thrust Axes and Arms/2(matrixOfJetsArms) -> matrixOfJetsArms/1
  Thrust Axes and Arms/1(matrixOfJetsAxes) -> matrixOfJetsAxes/1
  Pose Jet 4/1 -> Thrust Axes and Arms/4(w_H_J4)
  Pose Jet 3/1 -> Thrust Axes and Arms/3(w_H_J3)
  Pose Jet 1/1 -> Thrust Axes and Arms/1(w_H_J1)
  jointPos/1 -> Pose Jet 4/2, Pose Jet 3/2, Pose Jet 2/2, Pose Jet 1/2
  Pose Jet 2/1 -> Thrust Axes and Arms/2(w_H_J2)

== system momentumBasedFlight/FLIGHT CONTROLLER (CORE) V3.0/Flight Controller RAL-HUMANOIDS V3.0/Joint Torque Control for Flying/Integrate Joints Velocity error ==
  jointVel_err : Inport
  Constant : Constant  Value=zeros(Config.N_DOF,1)
  Discrete-Time Integrator1 : DiscreteIntegrator  InitialConditionSource=external  InitialCondition=zeros(Config.N_DOF,1)  SampleTime=Config.tStep  UpperSaturationLimit=20  LowerSaturationLimit=-20  ICPrevOutput=DiscIntNeverNeededParam  ICPrevScaledInput=DiscIntNeverNeededParam
  jointPos_err : Outport  VectorParamsAs1DForOutWhenUnconnected=off
  tag scope: jointPos_err_integral=global
  wires:
  Constant/1 -> Discrete-Time Integrator1/2
  jointVel_err/1 -> Discrete-Time Integrator1/1
  Discrete-Time Integrator1/1 -> [jointPos_err_integral], jointPos_err/1

== system momentumBasedFlight/FLIGHT CONTROLLER (CORE) V3.0/Flight Controller RAL-HUMANOIDS V3.0/Joint Torque Control for Flying/Plot Torque QP Residuals ==
  jointTorques_star : Inport
  contactForces_QP_star : Inport  Port=2
  sDDot_star : Inport  Port=3
  St_invM_B : Inport  Port=4
  St_invM_bias : Inport  Port=5
  Demux : Demux  Outputs=[3;3]
  Demux1 : Demux  Outputs=[3;3]
  Demux2 : Demux  Outputs=[6;6]
  Demux5 : Demux  Outputs=Config.numOfJointsForEachControlboard
  MATLAB Function : MATLAB Function  TreatAsAtomicUnit=on
  Sddot residuals : Scope  NumInputPorts=5
  left foot ext wrench : Scope  NumInputPorts=2
  right foot ext wrench : Scope  NumInputPorts=2
  wires:
  Demux1/1 -> right foot ext wrench/1  "linearForces"
  Demux2/1 -> Demux/1
  Demux5/2 -> Sddot residuals/2  "lArm"
  St_invM_bias/1 -> MATLAB Function/5(St_invM_bias)
  contactForces_QP_star/1 -> Demux2/1, MATLAB Function/2(contactForces_QP_star)
  Demux1/2 -> right foot ext wrench/2  "moments"
  St_invM_B/1 -> MATLAB Function/4(St_invM_B)
  jointTorques_star/1 -> MATLAB Function/1(jointTorques_star)
  Demux5/1 -> Sddot residuals/1  "torso"
  sDDot_star/1 -> MATLAB Function/3(sDDot_star)
  Demux2/2 -> Demux1/1
  Demux5/5 -> Sddot residuals/5  "rLeg"
  MATLAB Function/1(residual_sDDot) -> Demux5/1
  Demux5/4 -> Sddot residuals/4  "lLeg"
  Demux/2 -> left foot ext wrench/2  "moments"
  Demux5/3 -> Sddot residuals/3  "rArm"
  Demux/1 -> left foot ext wrench/1  "linearForces"

== system momentumBasedFlight/FLIGHT CONTROLLER (CORE) V3.0/Flight Controller RAL-HUMANOIDS V3.0/Joint Torque Control for Flying/QP torqueControl ==
  HessianMatrixQP : Inport
  gVectorQP : Inport  Port=2
  ConstraintMatrix_inequality : Inport  Port=3
  biasVectorConstraint_inequality : Inport  Port=4
  feetContactIsActive : Inport  Port=5
  Constant2 : Constant  Value=Config.sat.jointTorquesSaturation
  NOT : Logic  Operator=NOT  IconShape=distinctive  AllPortsSameDT=off  OutDataTypeStr=boolean
  Process QP Inputs Torque Control : MATLAB Function  TreatAsAtomicUnit=on
  QP torqueControl - balancing : Subsystem  TreatAsAtomicUnit=on
  QP torqueControl - flight : Subsystem  TreatAsAtomicUnit=on
  Select QP torqueControl Output : Subsystem
  jointTorques_star : Outport  VectorParamsAs1DForOutWhenUnconnected=off
  exitFlagQP_torqueControl : Outport  Port=2  VectorParamsAs1DForOutWhenUnconnected=off
  contactForces_QP_star : Outport  Port=3  VectorParamsAs1DForOutWhenUnconnected=off
  wires:
  Select QP torqueControl Output/1(jointTorques_star) -> jointTorques_star/1
  Select QP torqueControl Output/2(exitFlagQP_torqueControl) -> exitFlagQP_torqueControl/1
  QP torqueControl - flight/1(QPStatus_flight) -> Select QP torqueControl Output/4(QPStatus_flight)
  QP torqueControl - flight/2(QPOutput_flight) -> Select QP torqueControl Output/5(QPOutput_flight)
  QP torqueControl - balancing/2(QPOutput_balancing) -> Select QP torqueControl Output/2(QPOutput_balancing)
  QP torqueControl - balancing/1(QPStatus_balancing) -> Select QP torqueControl Output/1(QPStatus_balancing)
  Process QP Inputs Torque Control/1(H_balancing) -> QP torqueControl - balancing/1(H)
  Process QP Inputs Torque Control/2(g_balancing) -> QP torqueControl - balancing/2(g)
  Process QP Inputs Torque Control/3(ub_balancing) -> QP torqueControl - balancing/3(ub)
  Process QP Inputs Torque Control/4(lb_balancing) -> QP torqueControl - balancing/4(lb)
  Process QP Inputs Torque Control/5(Aeq_balancing) -> QP torqueControl - balancing/5(AEq)
  Process QP Inputs Torque Control/6(lbEq_balancing) -> QP torqueControl - balancing/6(lbEq)
  Process QP Inputs Torque Control/7(ubEq_balancing) -> QP torqueControl - balancing/7(ubEq)
  Process QP Inputs Torque Control/11(lb_flight) -> QP torqueControl - flight/4(lb)
  Process QP Inputs Torque Control/10(ub_flight) -> QP torqueControl - flight/3(ub)
  Process QP Inputs Torque Control/9(g_flight) -> QP torqueControl - flight/2(g)
  Process QP Inputs Torque Control/8(H_flight) -> QP torqueControl - flight/1(H)
  Constant2/1 -> Process QP Inputs Torque Control/5(jointTorquesSaturation)
  gVectorQP/1 -> Process QP Inputs Torque Control/2(gVectorQP)
  HessianMatrixQP/1 -> Process QP Inputs Torque Control/1(HessianMatrixQP)
  ConstraintMatrix_inequality/1 -> Process QP Inputs Torque Control/3(InequalityConstrMatrix)
  biasVectorConstraint_inequality/1 -> Process QP Inputs Torque Control/4(biasVectorInequalityConstr)
  NOT/1 -> QP torqueControl - flight/Enable
  feetContactIsActive/1 -> NOT/1, QP torqueControl - balancing/Enable, Select QP torqueControl Output/3(feetContactIsActive)
  Select QP torqueControl Output/3(contactForces_QP_star) -> contactForces_QP_star/1

== system momentumBasedFlight/FLIGHT CONTROLLER (CORE) V3.0/Flight Controller RAL-HUMANOIDS V3.0/Joint Torque Control for Flying/Torque Derivative Saturation ==
  jointTorques_star : Inport
  Constant1 : Constant  Value=Config.tStep
  Constant2 : Constant  Value=Config.sat.jointTorquesDotMax
  Saturate Torque Derivative : MATLAB Function  TreatAsAtomicUnit=on
  "holder " : WBToolboxLibrary/Utilities/holder 
      settings: SourceProductName=WholeBodyToolbox
  jointTorques_star_sat : Outport  VectorParamsAs1DForOutWhenUnconnected=off
  wires:
  Constant2/1 -> Saturate Torque Derivative/4(uDotMax)
  Constant1/1 -> Saturate Torque Derivative/3(tStep)
  "holder "/1 -> Saturate Torque Derivative/2(u_0)
  Saturate Torque Derivative/1(uSat) -> jointTorques_star_sat/1
  jointTorques_star/1 -> Saturate Torque Derivative/1(u), "holder "/1

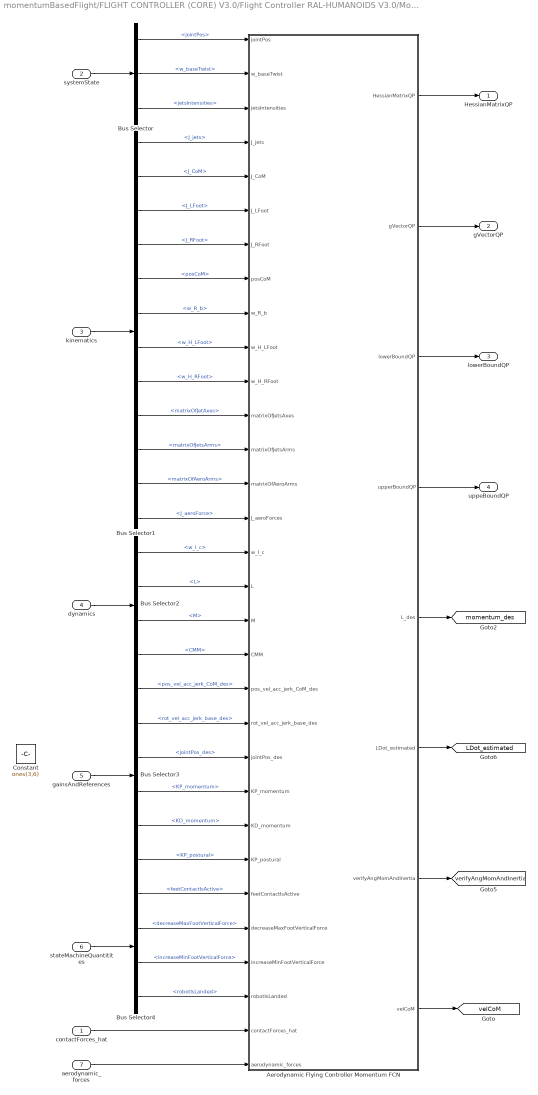
== system momentumBasedFlight/FLIGHT CONTROLLER (CORE) V3.0/Flight Controller RAL-HUMANOIDS V3.0/Momentum Control for Flying/Momentum Control ==
  contactForces_hat : Inport
  systemState : Inport  Port=2
  kinematics : Inport  Port=3
  dynamics : Inport  Port=4
  gainsAndReferences : Inport  Port=5
  stateMachineQuantitites : Inport  Port=6
  aerodynamic_forces : Inport  Port=7
  "Aerodynamic Flying Controller Momentum FCN " : MATLAB Function  TreatAsAtomicUnit=on
  Bus Selector : BusSelector  OutputSignals=jointPos,w_baseTwist,jetsIntensities
  Bus Selector1 : BusSelector  OutputSignals=J_jets,J_CoM,J_LFoot,J_RFoot,posCoM,w_R_b,w_H_LFoot,w_H_RFoot,matrixOfJetAxes,matrixOfJetsArms,matrixOfAeroArms,J_aeroForce
  Bus Selector2 : BusSelector  OutputSignals=w_I_c,L,M,CMM
  Bus Selector3 : BusSelector  OutputSignals=pos_vel_acc_jerk_CoM_des,rot_vel_acc_jerk_base_des,jointPos_des,KP_momentum,KD_momentum,KP_postural
  Bus Selector4 : BusSelector  OutputSignals=feetContactIsActive,decreaseMaxFootVerticalForce,increaseMinFootVerticalForce,robotIsLanded
  Constant : Constant  Value=ones(3,6)
  HessianMatrixQP : Outport  VectorParamsAs1DForOutWhenUnconnected=off
  gVectorQP : Outport  Port=2  VectorParamsAs1DForOutWhenUnconnected=off
  lowerBoundQP : Outport  Port=3  VectorParamsAs1DForOutWhenUnconnected=off
  uppeBoundQP : Outport  Port=4  VectorParamsAs1DForOutWhenUnconnected=off
  tag scope: LDot_estimated=global, momentum_des=global, velCoM=global, verifyAngMomAndInertia=global
  wires:
  "Aerodynamic Flying Controller Momentum FCN "/8(velCoM) -> [velCoM]
  contactForces_hat/1 -> "Aerodynamic Flying Controller Momentum FCN "/30(contactForces_hat)
  Bus Selector4/4 -> "Aerodynamic Flying Controller Momentum FCN "/29(robotIsLanded)  "<robotIsLanded>"
  Bus Selector4/3 -> "Aerodynamic Flying Controller Momentum FCN "/28(increaseMinFootVerticalForce)  "<increaseMinFootVerticalForce>"
  Bus Selector4/2 -> "Aerodynamic Flying Controller Momentum FCN "/27(decreaseMaxFootVerticalForce)  "<decreaseMaxFootVerticalForce>"
  Bus Selector2/1 -> "Aerodynamic Flying Controller Momentum FCN "/16(w_I_c)  "<w_I_c>"
  Bus Selector1/10 -> "Aerodynamic Flying Controller Momentum FCN "/13(matrixOfJetsArms)  "<matrixOfJetsArms>"
  Bus Selector1/9 -> "Aerodynamic Flying Controller Momentum FCN "/12(matrixOfJetsAxes)  "<matrixOfJetAxes>"
  Bus Selector3/1 -> "Aerodynamic Flying Controller Momentum FCN "/20(pos_vel_acc_jerk_CoM_des)  "<pos_vel_acc_jerk_CoM_des>"
  Bus Selector1/6 -> "Aerodynamic Flying Controller Momentum FCN "/9(w_R_b)  "<w_R_b>"
  Bus Selector1/5 -> "Aerodynamic Flying Controller Momentum FCN "/8(posCoM)  "<posCoM>"
  "Aerodynamic Flying Controller Momentum FCN "/5(L_des) -> [momentum_des]
  Bus Selector3/6 -> "Aerodynamic Flying Controller Momentum FCN "/25(KP_postural)  "<KP_postural>"
  Bus Selector2/2 -> "Aerodynamic Flying Controller Momentum FCN "/17(L)  "<L>"
  Bus Selector1/7 -> "Aerodynamic Flying Controller Momentum FCN "/10(w_H_LFoot)  "<w_H_LFoot>"
  Bus Selector3/5 -> "Aerodynamic Flying Controller Momentum FCN "/24(KD_momentum)  "<KD_momentum>"
  "Aerodynamic Flying Controller Momentum FCN "/6(LDot_estimated) -> [LDot_estimated]
  Bus Selector2/3 -> "Aerodynamic Flying Controller Momentum FCN "/18(M)  "<M>"
  Bus Selector2/4 -> "Aerodynamic Flying Controller Momentum FCN "/19(CMM)  "<CMM>"
  Bus Selector1/8 -> "Aerodynamic Flying Controller Momentum FCN "/11(w_H_RFoot)  "<w_H_RFoot>"
  Bus Selector1/4 -> "Aerodynamic Flying Controller Momentum FCN "/7(J_RFoot)  "<J_RFoot>"
  Bus Selector/3 -> "Aerodynamic Flying Controller Momentum FCN "/3(jetsIntensities)  "<jetsIntensities>"
  gainsAndReferences/1 -> Bus Selector3/1
  Bus Selector1/2 -> "Aerodynamic Flying Controller Momentum FCN "/5(J_CoM)  "<J_CoM>"
  dynamics/1 -> Bus Selector2/1
  Bus Selector3/4 -> "Aerodynamic Flying Controller Momentum FCN "/23(KP_momentum)  "<KP_momentum>"
  "Aerodynamic Flying Controller Momentum FCN "/3(lowerBoundQP) -> lowerBoundQP/1
  stateMachineQuantitites/1 -> Bus Selector4/1
  "Aerodynamic Flying Controller Momentum FCN "/7(verifyAngMomAndInertia) -> [verifyAngMomAndInertia]
  Bus Selector4/1 -> "Aerodynamic Flying Controller Momentum FCN "/26(feetContactIsActive)  "<feetContactIsActive>"
  "Aerodynamic Flying Controller Momentum FCN "/2(gVectorQP) -> gVectorQP/1
  "Aerodynamic Flying Controller Momentum FCN "/4(upperBoundQP) -> uppeBoundQP/1
  "Aerodynamic Flying Controller Momentum FCN "/1(HessianMatrixQP) -> HessianMatrixQP/1
  Bus Selector/2 -> "Aerodynamic Flying Controller Momentum FCN "/2(w_baseTwist)  "<w_baseTwist>"
  Bus Selector1/1 -> "Aerodynamic Flying Controller Momentum FCN "/4(J_jets)  "<J_jets>"
  Bus Selector/1 -> "Aerodynamic Flying Controller Momentum FCN "/1(jointPos)  "<jointPos>"
  kinematics/1 -> Bus Selector1/1
  Bus Selector1/3 -> "Aerodynamic Flying Controller Momentum FCN "/6(J_LFoot)  "<J_LFoot>"
  Bus Selector3/3 -> "Aerodynamic Flying Controller Momentum FCN "/22(jointPos_des)  "<jointPos_des>"
  systemState/1 -> Bus Selector/1
  Bus Selector3/2 -> "Aerodynamic Flying Controller Momentum FCN "/21(rot_vel_acc_jerk_base_des)  "<rot_vel_acc_jerk_base_des>"
  aerodynamic_forces/1 -> "Aerodynamic Flying Controller Momentum FCN "/31(aerodynamic_forces)
  Bus Selector1/11 -> "Aerodynamic Flying Controller Momentum FCN "/14(matrixOfAeroArms)  "<matrixOfAeroArms>"
  Bus Selector1/12 -> "Aerodynamic Flying Controller Momentum FCN "/15(J_aeroForces)  "<J_aeroForce>"
